simulink model "untitled1"  (Simulink 7.9)
settings: Solver=ode45  StartTime=0.0  StopTime=30  RelTol=1e-3
settings Model: Creator=sony  LastModifiedBy=sony

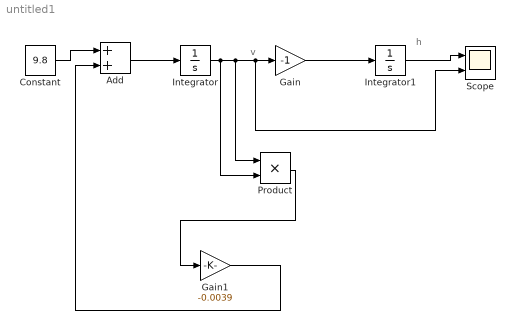
== system untitled1 ==
  note: h
  note: v
  Add : Sum
  Constant : Constant  Value=9.8
  Gain : Gain  Gain=-1
  Gain1 : Gain  Gain=-0.0039
  Integrator : Integrator
  Integrator1 : Integrator  InitialCondition=1000
  Product : Product  RndMeth=Zero
  Scope : Scope  NumInputPorts=2
      settings: RequirementInfo="{}  %GIDa_0884e69a_bfd3_463e_9caa_98d651a3ae66"  TimeRange=30  YMin=-1000~0  YMax=1000~100
  wires:
  Integrator/1 -> Product/1, Gain/1, Scope/2, Product/2
  Gain/1 -> Integrator1/1
  Integrator1/1 -> Scope/1
  Product/1 -> Gain1/1
  Gain1/1 -> Add/2
  Constant/1 -> Add/1
  Add/1 -> Integrator/1
